simulink model "fir_model"  (R2020b)
settings: Solver=VariableStepAuto  StartTime=0.0  StopTime=1  RelTol=1e-3
settings Model: Creator=pablo  LastModifiedBy=pablo

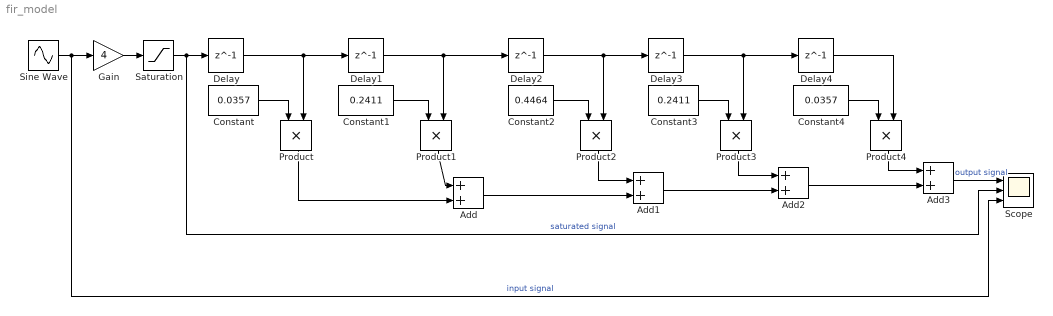
== system fir_model ==
  Add{,1..3} (4 alike) : Sum
  Constant : Constant  Value=0.0357
  Constant1 : Constant  Value=0.2411
  Constant2 : Constant  Value=0.4464
  Constant3 : Constant  Value=0.2411
  Constant4 : Constant  Value=0.0357
  Delay{,1..4} (5 alike) : Delay  DelayLength=1  InitialCondition=0  SampleTime=1e-4
  Gain : Gain  Gain=4
  Product{,1..4} (5 alike) : Product
  Saturation : Saturate  UpperLimit=1  LowerLimit=-1
  Scope : Scope  NumInputPorts=3
  Sine Wave : Sin  SineType=Sample based  Amplitude=2  Samples=20  SampleTime=1e-4
  wires:
  Delay/1 -> Product/2, Delay1/1
  Delay1/1 -> Delay2/1, Product1/2
  Delay2/1 -> Delay3/1, Product2/2
  Delay3/1 -> Product3/2, Delay4/1
  Product1/1 -> Add/1
  Product/1 -> Add/2
  Product2/1 -> Add1/1
  Add/1 -> Add1/2
  Product3/1 -> Add2/1
  Add1/1 -> Add2/2
  Constant/1 -> Product/1
  Constant1/1 -> Product1/1
  Constant2/1 -> Product2/1
  Constant3/1 -> Product3/1
  Saturation/1 -> Scope/2, Delay/1  "saturated signal"
  Sine Wave/1 -> Gain/1, Scope/3  "input signal"
  Product4/1 -> Add3/1
  Constant4/1 -> Product4/1
  Delay4/1 -> Product4/2
  Add2/1 -> Add3/2
  Add3/1 -> Scope/1  "output signal"
  Gain/1 -> Saturation/1
